simulink subsystem "ACDCConveter"  (R2024a)
settings: Solver=VariableStepAuto  StartTime=0.0  StopTime=1.5  RelTol=1e-3
undefined symbols (not defined in the file): D1, Delta, DiscIntNeverNeededParam, Ts_Control, Ts_Power
libraries: spsSeriesRLCBranchLib x5, spsSecondOrderFilterLib x3, spsThreePhaseSeriesRLCLoadLib x2, spsMeanLib x2, spsabctodq0Lib x2, spsVoltageMeasurementLib x2, spsStairGeneratorLib x1, spsThreePhaseVIMeasurementLib x1, spsPLL3phLib x1, simulink_extras x1, spsPWMGenerator3LevelLib x1, spsGroundLib x1
settings Model: DefaultTestHarness=ACDCConveter_Harness1  Creator=nakamura  LastModifiedBy=nakamura

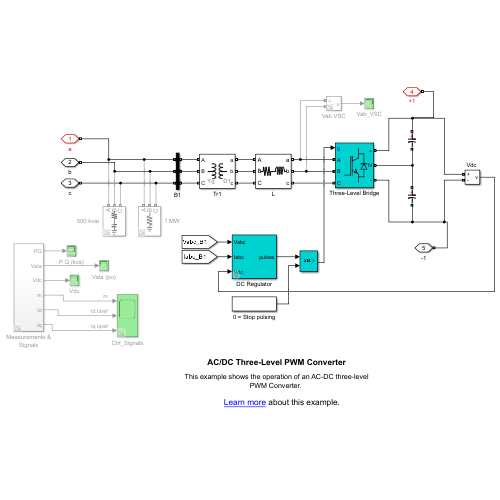
[thumbnail: Simulink's stored preview of the top-level diagram]
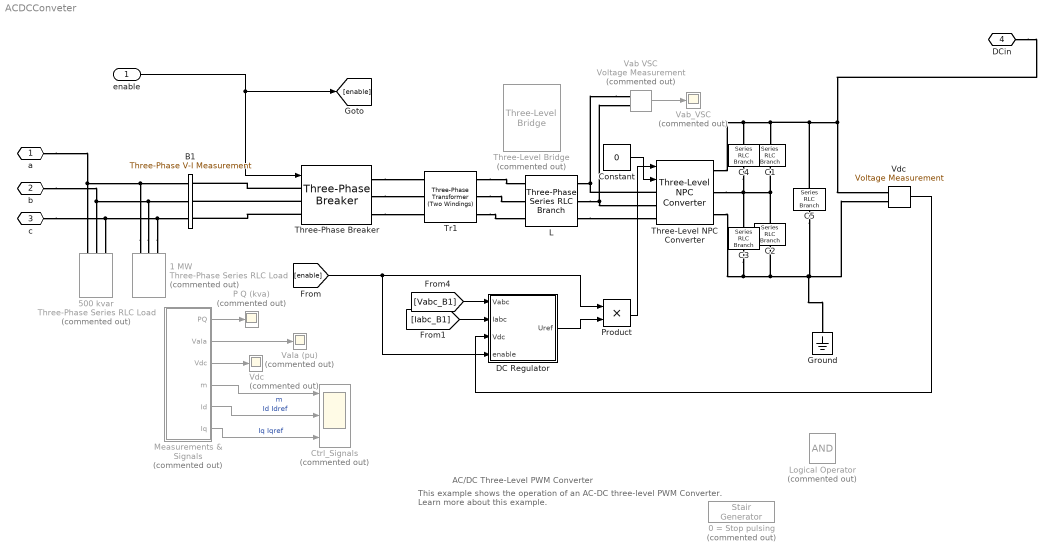
== system ACDCConveter ==
  note: AC/DC Three-Level PWM Converter
  note: This example shows the operation of an AC-DC three-level PWM Converter.
      |
      | Learn more about this example.
  enable : Inport
  0 = Stop pulsing : spsStairGeneratorLib/Stair Generator  Commented=on  t=[0 0.1]*10000000  e=[1 0]  Ts=Ts_Power
  1 MW : spsThreePhaseSeriesRLCLoadLib/Three-Phase Series RLC Load  Commented=on  LConnTagsString=A|B|C  Configuration=Y (grounded)  NominalVoltage=600  Vabc=[1e3 1e3 1e3]  Vabcp=[1e3 1e3 1e3]  NominalFrequency=60  UnbalancedPower=off  ActivePower=1e6  InductivePower=0  CapacitivePower=0  Pabc=[10e3 9e3 11e3]  QLabc=[100 90 110]  QCabc=[100 90 110]  Pabcp=[10e3 9e3 11e3]  QLabcp=[100 90 110]  QCabcp=[100 90 110]  Measurements=None  LoadType=constant Z
  500 kvar : spsThreePhaseSeriesRLCLoadLib/Three-Phase Series RLC Load  Commented=on  LConnTagsString=A|B|C  Configuration=Y (grounded)  NominalVoltage=600  Vabc=[1e3 1e3 1e3]  Vabcp=[1e3 1e3 1e3]  NominalFrequency=60  UnbalancedPower=off  ActivePower=0.5e6/100  InductivePower=0  CapacitivePower=0.5e6  Pabc=[10e3 9e3 11e3]  QLabc=[100 90 110]  QCabc=[100 90 110]  Pabcp=[10e3 9e3 11e3]  QLabcp=[100 90 110]  QCabcp=[100 90 110]  Measurements=None  LoadType=constant Z
  B1 : spsThreePhaseVIMeasurementLib/Three-Phase V-I Measurement  VoltageMeasurement=phase-to-ground  SetLabelV=on  LabelV=Vabc_B1  Vpu=off  VpuLL=off  CurrentMeasurement=yes  SetLabelI=on  LabelI=Iabc_B1  Ipu=off  Pbase=100e6  Vbase=500e3  OutputType=Magnitude  PhasorSimulation=off  PSBequivalent=0
  C1 : spsSeriesRLCBranchLib/Series RLC Branch  LConnTagsString=__new0  RConnTagsString=__new0  BranchType=C  Resistance=1.0  Inductance=1.0  SetiL0=off  InitialCurrent=0  Capacitance=75000e-06  Setx0=off  InitialVoltage=0  Measurements=None
  C2 : spsSeriesRLCBranchLib/Series RLC Branch  LConnTagsString=__new0  RConnTagsString=__new0  BranchType=C  Resistance=1.0  Inductance=1.0  SetiL0=off  InitialCurrent=0  Capacitance=75000e-06  Setx0=off  InitialVoltage=0  Measurements=None
  C3 : spsSeriesRLCBranchLib/Series RLC Branch  LConnTagsString=__new0  RConnTagsString=__new0  BranchType=R  Resistance=1e8  Inductance=1.0  SetiL0=off  InitialCurrent=0  Capacitance=75000e-06  Setx0=off  InitialVoltage=0  Measurements=None
  C4 : spsSeriesRLCBranchLib/Series RLC Branch  LConnTagsString=__new0  RConnTagsString=__new0  BranchType=R  Resistance=1e8  Inductance=1.0  SetiL0=off  InitialCurrent=0  Capacitance=75000e-06  Setx0=off  InitialVoltage=0  Measurements=None
  C5 : spsSeriesRLCBranchLib/Series RLC Branch  LConnTagsString=__new0  RConnTagsString=__new0  BranchType=C  Resistance=1.0  Inductance=1.0  SetiL0=off  InitialCurrent=0  Capacitance=1e-03  Setx0=off  InitialVoltage=0  Measurements=None
  Constant : Constant  Value=0
  Ctrl_Signals : Scope  Commented=on  NumInputPorts=3
  DC Regulator : Subsystem  mask(DC Voltage Regulator){Vdc_Ref=450}
      mask prompts: Vdc_Ref "DC voltage setpoint (V):"
  Ground : spsGroundLib/Ground  LConnTagsString=a
  L : spsThreePhaseSeriesRLCBranchLib/Three-Phase Series RLC Branch  LConnTagsString=A|B|C  RConnTagsString=A|B|C  BranchType=RL  Resistance=0.1e-3  Inductance=20e-6  Capacitance=inf  Measurements=None
  Logical Operator : Logic  Commented=on  AllPortsSameDT=off  OutDataTypeStr=float('double')
  Measurements & Signals : Subsystem  Commented=on
  P Q (kva) : Scope  Commented=on
  Product : Product
  Three-Level NPC Converter : spsThreeLevelNPCConverterLib/Three-Level NPC Converter  ModelType=Average model (Uref-controlled)  Ron=1e-7  Rs=1e6  Cs=inf  Vforward=[0,0]  Ron_Diode=1e-6  Rs_Diode=1e6  Cs_Diode=inf  Vf_Diode=0  Rs_CurrentSource=inf  Ron_ACsource=1e-10
  Three-Level Bridge : spsThreeLevelBridgeLib/Three-Level Bridge  Commented=on  Arms=3  SnubberResistance=50  SbubberCapacitance=1e-6  Device=IGBT / Diodes  Ron=0.2e-3  ForwardVoltages="[  2 1 ]"  Measurements=All voltages and currents
      settings: AttributesFormatString=\n
  Three-Phase Breaker : spsThreePhaseBreakerLib/Three-Phase Breaker  InitialState=open  SwitchA=on  SwitchB=on  SwitchC=on  SwitchTimes="[1/60  5/60]"  External=on  BreakerResistance=1e-6  SnubberResistance=1e7  SnubberCapacitance=inf  Measurements=None
  Tr1 : spsThreePhaseTransformerTwoWindingsLib/Three-Phase Transformer (Two Windings)  Winding1Connection=Yg  Winding2Connection=Delta (D1)  CoreType=Three single-phase transformers  SetSaturation=off  Hysteresis=off  DataFile='hysteresis'  SetInitialFlux=off  Measurements=None  UNITS=pu  NominalPower=[ 500e3 , 60 ]  Winding1=[ 6.6e3 , 0.04/30/2 , 0.04 ]  Winding2=[ 210 , 0.04/30/2 , 0.0 ]  Rm=500  Lm=500  L0=0.5  Saturation=[ 0,0 ; 0.0024,1.2 ; 1.0,1.52 ]  InitialFluxes=[ 0.8 , -0.8 , 0.7 ]  BreakLoop=off  DiscreteSolver=Trapezoidal iterative  DataType=off  TransfoNumber=0
  VaIa (pu) : Scope  Commented=on
  Vab VSC : spsVoltageMeasurementLib/Voltage Measurement  Tag=PoWeRsYsTeMmEaSuReMeNt  Commented=on  PhasorSimulation=off  OutputType=Magnitude  PSBequivalent=0
  Vab_VSC : Scope  Commented=on
  Vdc : Scope  Commented=on
  "Vdc " : spsVoltageMeasurementLib/Voltage Measurement  Tag=PoWeRsYsTeMmEaSuReMeNt  PhasorSimulation=off  OutputType=Magnitude  PSBequivalent=0
  a : PMIOPort  Side=Left
  b : PMIOPort  Port=2  Side=Left
  c : PMIOPort  Port=3  Side=Left
  DCin : PMIOPort  Port=4  Side=Right
  wires:
  Measurements & Signals/5(Id) -> Ctrl_Signals/2  "Id Idref"
  Measurements & Signals/6(Iq) -> Ctrl_Signals/3  "Iq Iqref"
  [Iabc_B1] -> DC Regulator/2(Iabc)
  Measurements & Signals/4(m) -> Ctrl_Signals/1  "m"
  Measurements & Signals/1(PQ) -> P Q (kva)/1
  Vab VSC/1 -> Vab_VSC/1
  Measurements & Signals/2(VaIa) -> VaIa (pu)/1
  [Vabc_B1] -> DC Regulator/1(Vabc)
  "Vdc "/1 -> DC Regulator/3(Vdc)
  Measurements & Signals/3(Vdc) -> Vdc/1
  Constant/1 -> Three-Level NPC Converter/2
  Product/1 -> Three-Level NPC Converter/1
  enable/1 -> [enable], Three-Phase Breaker/1
  [enable] -> Product/1, DC Regulator/4(enable)
  DC Regulator/1(Uref) -> Product/2
  connections:
  1 MW/LConn1 -- a/RConn1 -- 500 kvar/LConn1 -- B1/LConn1
  C5/RConn1 -- "Vdc "/LConn2 -- Ground/LConn1 -- Three-Level NPC Converter/RConn3 -- C3/RConn1 -- C2/RConn1
  Three-Level NPC Converter/RConn1 -- C4/LConn1 -- C1/LConn1 -- C5/LConn1 -- "Vdc "/LConn1 -- DCin/RConn1
  C2/LConn1 -- Three-Level NPC Converter/RConn2 -- C4/RConn1 -- C3/LConn1 -- C1/RConn1
  1 MW/LConn3 -- c/RConn1 -- 500 kvar/LConn3 -- B1/LConn3
  1 MW/LConn2 -- b/RConn1 -- 500 kvar/LConn2 -- B1/LConn2
  L/RConn2 -- Vab VSC/LConn2 -- Three-Level NPC Converter/LConn2
  Vab VSC/LConn1 -- Three-Level NPC Converter/LConn1 -- L/RConn1
  Three-Phase Breaker/LConn2 -- B1/RConn2
  Three-Phase Breaker/LConn3 -- B1/RConn3
  Tr1/RConn1 -- L/LConn1
  Three-Phase Breaker/LConn1 -- B1/RConn1
  Tr1/RConn3 -- L/LConn3
  L/RConn3 -- Three-Level NPC Converter/LConn3
  Tr1/RConn2 -- L/LConn2
  Three-Phase Breaker/RConn1 -- Tr1/LConn1
  Three-Phase Breaker/RConn2 -- Tr1/LConn2
  Three-Phase Breaker/RConn3 -- Tr1/LConn3

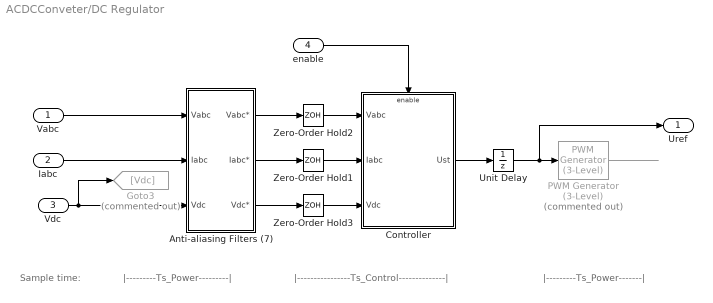
== system ACDCConveter/DC Regulator ==
  note: |----------------Ts_Control--------------|
  note: |---------Ts_Power---------|
  note: Sample time:
  note: |---------Ts_Power-------|
  Vabc : Inport  PortDimensions=3
  Iabc : Inport  Port=2  PortDimensions=3
  Vdc : Inport  Port=3  PortDimensions=1
  enable : Inport  Port=4  PortDimensions=1
  Anti-aliasing Filters (7) : Subsystem  mask(Anti-aliasing (2nd order lowpass)){Fc=750, Ts=Ts_Power}
      mask prompts: Fc "Cut-off frequency (Hz):"; Ts "Sample time:"
  Controller : Subsystem  mask(DC Regulator){Vdc_Ref=Vdc_Ref, Par_VdcReg=[0.015 1.6], Par_IReg=[0.3 20], Par_Nom=[6.6e3 500e3], Ts=Ts_Control}
      mask prompts: Vdc_Ref "DC Voltage setpoint (Volts)"; Par_VdcReg "Vdc Regulator Gains: [ Kp  Ki ]"; Par_IReg "Current Regulators Gain: [ Kp Ki Kd ]"; Par_Nom "Nominal Voltage and power: [ Vnom (volts rms L-L)  Pnom (VA) ]"; Ts "Time Step (s)"
      mask init:
      | Vnom=Par_Nom(1);
      | Pnom=Par_Nom(2);
      | Kp_I=Par_IReg(1);
      | Ki_I=Par_IReg(2);
      | Kp_Vdc=Par_VdcReg(1);
      | Ki_Vdc=Par_VdcReg(2);
  Goto3 : Goto  Commented=on  GotoTag=Vdc
  PWM Generator (3-Level) : spsPWMGenerator3LevelLib/PWM Generator (3-Level)  Commented=on  ModulatorType=Three-phase bridge (12 pulses)  ModulatorMode=Unsynchronized  nF=27  Fc=27*60  ModulatingSignals=off  m=0.8  Freq=60  Phase=0  Ts=Ts_Power
  Unit Delay : UnitDelay  SampleTime=Ts_Control  HasFrameUpgradeWarning=on
  Zero-Order Hold1 : ZeroOrderHold  SampleTime=Ts_Control
  Zero-Order Hold2 : ZeroOrderHold  SampleTime=Ts_Control
  Zero-Order Hold3 : ZeroOrderHold  SampleTime=Ts_Control
  Uref : Outport  VectorParamsAs1DForOutWhenUnconnected=off
  wires:
  enable/1 -> Controller/Enable
  PWM Generator (3-Level)/1 -> ?
  Unit Delay/1 -> PWM Generator (3-Level)/1, Uref/1
  Controller/1(Ust) -> Unit Delay/1
  Anti-aliasing Filters (7)/1(" Vabc*") -> Zero-Order Hold2/1
  Anti-aliasing Filters (7)/2(Iabc*) -> Zero-Order Hold1/1
  Anti-aliasing Filters (7)/3(" Vdc*") -> Zero-Order Hold3/1
  Zero-Order Hold3/1 -> Controller/3(Vdc)
  Zero-Order Hold1/1 -> Controller/2(Iabc)
  Zero-Order Hold2/1 -> Controller/1(Vabc)
  Vdc/1 -> Goto3/1, Anti-aliasing Filters (7)/3("Vdc ")
  Iabc/1 -> Anti-aliasing Filters (7)/2("Iabc ")
  Vabc/1 -> Anti-aliasing Filters (7)/1(Vabc)

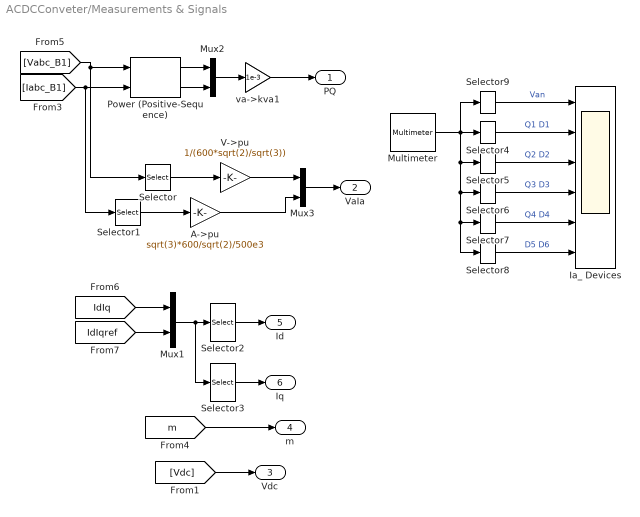
== system ACDCConveter/Measurements & Signals ==
  A->pu : Gain  Gain=sqrt(3)*600/sqrt(2)/500e3  SaturateOnIntegerOverflow=on  OutDataTypeStr=Inherit: Same as input  ParamDataTypeStr=Inherit: Same as input
  Ia_ Devices : Scope  NumInputPorts=6
  Multimeter : spsMultimeterLib/Multimeter  Tag=PoWeRsYsTeMmEaSuReMeNt  L=35  sel=[1 6 7 8 9 10 11 12 13 14 15]  yselected={}  Gain=[1 1 1 1 1 1 1 1 1 1 1]  OutputType=Magnitude  PlotAtSimulationStop=off  PhasorSimulation=off
      settings: AttributesFormatString=\n
  Mux1 : Mux  Inputs=2
  Mux2 : Mux  Inputs=2
  Mux3 : Mux  Inputs=2
  Power (Positive-Sequence) : spsPowerPositiveSequenceLib/Power (Positive-Sequence)  Freq=60  Vinit=[370 0]  Iinit=[5 0]  Ts=Ts_Power
  Selector : Selector  InputPortWidth=3  IndexOptions=Index vector (dialog)  Indices=1  OutputSizes=1
  Selector1 : Selector  InputPortWidth=3  IndexOptions=Index vector (dialog)  Indices=1  OutputSizes=1
  Selector2 : Selector  InputPortWidth=4  IndexOptions=Index vector (dialog)  Indices=[1 3]  OutputSizes=1
  Selector3 : Selector  InputPortWidth=4  IndexOptions=Index vector (dialog)  Indices=[1 3]+1  OutputSizes=1
  Selector4 : Selector  InputPortWidth=11  IndexOptions=Index vector (dialog)  Indices=[1 5]+1  OutputSizes=1
  Selector5 : Selector  InputPortWidth=11  IndexOptions=Index vector (dialog)  Indices=[1 5]+2  OutputSizes=1
  Selector6 : Selector  InputPortWidth=11  IndexOptions=Index vector (dialog)  Indices=[1 5]+3  OutputSizes=1
  Selector7 : Selector  InputPortWidth=11  IndexOptions=Index vector (dialog)  Indices=[1 5]+4  OutputSizes=1
  Selector8 : Selector  InputPortWidth=11  IndexOptions=Index vector (dialog)  Indices=[10 11]  OutputSizes=1
  Selector9 : Selector  InputPortWidth=11  IndexOptions=Index vector (dialog)  Indices=1  OutputSizes=1
  V->pu : Gain  Gain=1/(600*sqrt(2)/sqrt(3))  SaturateOnIntegerOverflow=on  OutDataTypeStr=Inherit: Same as input  ParamDataTypeStr=Inherit: Same as input
  va->kva1 : Gain  Gain=1e-3  SaturateOnIntegerOverflow=on  OutDataTypeStr=Inherit: Same as input  ParamDataTypeStr=Inherit: Same as input
  PQ : Outport  VectorParamsAs1DForOutWhenUnconnected=off
  VaIa : Outport  Port=2  VectorParamsAs1DForOutWhenUnconnected=off
  Vdc : Outport  Port=3  VectorParamsAs1DForOutWhenUnconnected=off
  m : Outport  Port=4  VectorParamsAs1DForOutWhenUnconnected=off
  Id : Outport  Port=5  VectorParamsAs1DForOutWhenUnconnected=off
  Iq : Outport  Port=6  VectorParamsAs1DForOutWhenUnconnected=off
  wires:
  Selector8/1 -> Ia_ Devices/6  "D5 D6"
  Selector7/1 -> Ia_ Devices/5  "Q4 D4"
  Selector6/1 -> Ia_ Devices/4  "Q3 D3"
  Selector5/1 -> Ia_ Devices/3  "Q2 D2"
  Selector4/1 -> Ia_ Devices/2  "Q1 D1"
  Selector9/1 -> Ia_ Devices/1  "Van"
  A->pu/1 -> Mux3/2
  V->pu/1 -> Mux3/1
  Selector3/1 -> Iq/1
  Selector2/1 -> Id/1
  [m] -> m/1
  Mux1/1 -> Selector3/1, Selector2/1
  [Vdc] -> Vdc/1
  Mux3/1 -> VaIa/1
  [Iabc_B1] -> Power (Positive-Sequence)/2, Selector1/1
  [Vabc_B1] -> Power (Positive-Sequence)/1, Selector/1
  Selector1/1 -> A->pu/1
  Selector/1 -> V->pu/1
  [IdIqref] -> Mux1/2
  [IdIq] -> Mux1/1
  Multimeter/1 -> Selector9/1, Selector8/1, Selector7/1, Selector6/1, Selector5/1, Selector4/1
  Power (Positive-Sequence)/1 -> Mux2/1
  Power (Positive-Sequence)/2 -> Mux2/2
  Mux2/1 -> va->kva1/1
  va->kva1/1 -> PQ/1

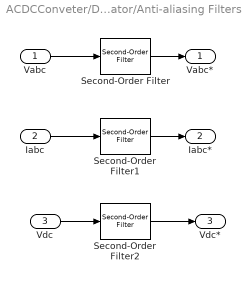
== system ACDCConveter/DC Regulator/Anti-aliasing Filters (7) ==
  Vabc : Inport  PortDimensions=3
  "Iabc " : Inport  Port=2  PortDimensions=3
  "Vdc " : Inport  Port=3  PortDimensions=1
  Second-Order Filter : spsSecondOrderFilterLib/Second-Order Filter  FilterType=Lowpass  Fo=Fc  Zeta=0.707  Ts=Ts  Initialize=off  Vac_Init="[0,  0,  60]"  Vdc_Init=0  PlotResponse=off  FreqRange=[0, 500, 1]
  Second-Order Filter1 : spsSecondOrderFilterLib/Second-Order Filter  FilterType=Lowpass  Fo=Fc  Zeta=0.707  Ts=Ts  Initialize=off  Vac_Init="[0,  0,  60]"  Vdc_Init=0  PlotResponse=off  FreqRange=[0, 500, 1]
  Second-Order Filter2 : spsSecondOrderFilterLib/Second-Order Filter  FilterType=Lowpass  Fo=Fc  Zeta=0.707  Ts=Ts  Initialize=off  Vac_Init="[0,  0,  60]"  Vdc_Init=0  PlotResponse=off  FreqRange=[0, 500, 1]
  " Vabc*" : Outport  VectorParamsAs1DForOutWhenUnconnected=off
  Iabc* : Outport  Port=2  VectorParamsAs1DForOutWhenUnconnected=off
  " Vdc*" : Outport  Port=3  VectorParamsAs1DForOutWhenUnconnected=off
  wires:
  Second-Order Filter2/1 -> " Vdc*"/1
  "Vdc "/1 -> Second-Order Filter2/1
  Vabc/1 -> Second-Order Filter/1
  Second-Order Filter/1 -> " Vabc*"/1
  "Iabc "/1 -> Second-Order Filter1/1
  Second-Order Filter1/1 -> Iabc*/1

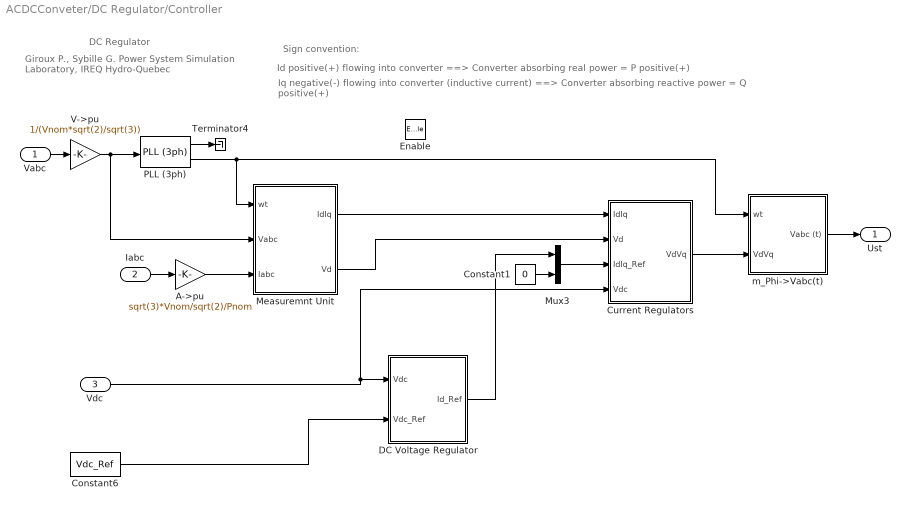
== system ACDCConveter/DC Regulator/Controller ==
  note: DC Regulator
  note: Giroux P., Sybille G.
      | Power System Simulation Laboratory, IREQ
      | Hydro-Quebec
  note: Iq negative(-) flowing into converter (inductive current) ==> Converter absorbing reactive power = Q positive(+)
  note: Sign convention:
  note: Id positive(+) flowing into converter ==> Converter absorbing real power = P positive(+)
  Vabc : Inport  PortDimensions=3
  Iabc : Inport  Port=2  PortDimensions=3
  Vdc : Inport  Port=3  PortDimensions=1
  Enable : EnablePort  StatesWhenEnabling=reset
  A->pu : Gain  Gain=sqrt(3)*Vnom/sqrt(2)/Pnom  SaturateOnIntegerOverflow=on  OutDataTypeStr=Inherit: Same as input  ParamDataTypeStr=Inherit: Same as input
  Constant1 : Constant  Value=0
  Constant6 : Constant  Value=Vdc_Ref
  Current Regulators : Subsystem  mask(Current Regulators){Kp=Kp_I, Ki=Ki_I, Kd=0, TcD=0.2e-3, Par_Limits=[12 -12], Init=0, Ts=Ts}
      mask prompts: Kp "Proportional gain (Kp):"; Ki "Integral gain (Ki):"; Kd "Derivative gain (Kd):"; TcD "Time constant for derivative (s):"; Par_Limits "Output limits: [ Upper   Lower ]"; Init "Output initial value:"; Ts "Sample time:"
      mask help:
      | Sign convention:
      | Id positive(+) flowing into converter ==> Converter absorbing real power = P positive(+)
      | Iq negative(-) flowing into converter (inductive current) ==> Converter absorbing reactive power = Q positive(+)
  DC Voltage Regulator : Subsystem  mask(DC Voltage regulator){Kp=Kp_Vdc, Ki=Ki_Vdc, Ts=Ts}
      mask prompts: Kp "Proportional gain (Kp):"; Ki "Integral gain(Ki)"; Ts "Sample time:"
  Measuremnt Unit : Subsystem
  Mux3 : Mux  Inputs=2
  PLL (3ph) : spsPLL3phLib/PLL (3ph)  Fmin=45  Par_Init=[-45 60]  ParK=[60 1400]  TcD=1e-4  MaxRateChangeFreq=12  FilterCutOffFreq=25  Ts=1e-5  AGC=off
  Terminator4 : Terminator
  V->pu : Gain  Gain=1/(Vnom*sqrt(2)/sqrt(3))  SaturateOnIntegerOverflow=on  OutDataTypeStr=Inherit: Same as input  ParamDataTypeStr=Inherit: Same as input
  m_Phi->Vabc(t) : Subsystem
  Ust : Outport  VectorParamsAs1DForOutWhenUnconnected=off
  wires:
  Constant6/1 -> DC Voltage Regulator/2(Vdc_Ref)
  m_Phi->Vabc(t)/1(Vabc (t)) -> Ust/1
  PLL (3ph)/2 -> m_Phi->Vabc(t)/1(wt), Measuremnt Unit/1(wt)
  Current Regulators/1(VdVq) -> m_Phi->Vabc(t)/2(VdVq)
  DC Voltage Regulator/1(Id_Ref) -> Mux3/1
  Constant1/1 -> Mux3/2
  Mux3/1 -> Current Regulators/3(IdIq_Ref)
  Measuremnt Unit/2(Vd) -> Current Regulators/2(Vd)
  Measuremnt Unit/1(IdIq) -> Current Regulators/1(IdIq)
  Iabc/1 -> A->pu/1
  PLL (3ph)/1 -> Terminator4/1
  Vdc/1 -> Current Regulators/4(Vdc), DC Voltage Regulator/1(Vdc)
  Vabc/1 -> V->pu/1
  V->pu/1 -> PLL (3ph)/1, Measuremnt Unit/2(Vabc)
  A->pu/1 -> Measuremnt Unit/3(Iabc)

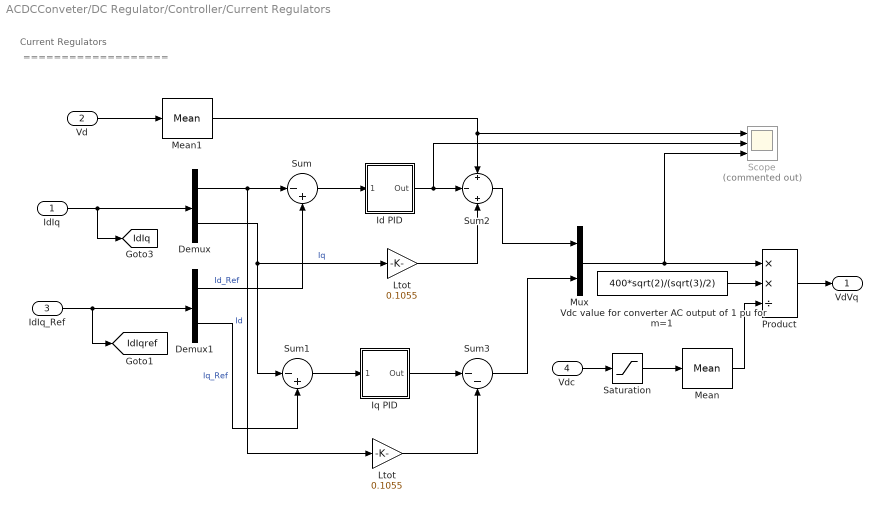
== system ACDCConveter/DC Regulator/Controller/Current Regulators ==
  note: ===================
  note: Current Regulators
  IdIq : Inport  PortDimensions=2
  Vd : Inport  Port=2
  IdIq_Ref : Inport  Port=3  PortDimensions=2
  Vdc : Inport  Port=4
  " Ltot" : Gain  Gain=0.1055  SaturateOnIntegerOverflow=on  OutDataTypeStr=Inherit: Same as input  ParamDataTypeStr=Inherit: Same as input
  Demux : Demux  Outputs=2
      settings: DisplayOption=none
  Demux1 : Demux  Outputs=2
      settings: DisplayOption=none
  Id PID : Subsystem  DialogController=POWERSYS.PowerSysDialog  mask(Discrete PID Controller){Kp=Kp, Ki=Ki, Kd=Kd, TcD=TcD, Par_Limits=Par_Limits, Init=Init, Ts=Ts}
      mask prompts: Kp "Proportional gain (Kp):"; Ki "Integral gain (Ki):"; Kd "Derivative gain (Kd):"; TcD "Time constant for derivative (s):"; Par_Limits "Output limits: [ Upper   Lower ]"; Init "Output initial value:"; Ts "Sample time:"
      mask help: This block implements a discrete PID controller.
      mask init:
      | UpperLimit=Par_Limits(1);
      | LowerLimit=Par_Limits(2);
      | power_initmask();
      mask Display: disp('PID');
  Iq PID : Subsystem  DialogController=POWERSYS.PowerSysDialog  mask(Discrete PID Controller){Kp=Kp, Ki=Ki, Kd=Kd, TcD=TcD, Par_Limits=Par_Limits, Init=Init, Ts=Ts}
      mask prompts: Kp "Proportional gain (Kp):"; Ki "Integral gain (Ki):"; Kd "Derivative gain (Kd):"; TcD "Time constant for derivative (s):"; Par_Limits "Output limits: [ Upper   Lower ]"; Init "Output initial value:"; Ts "Sample time:"
      mask help: This block implements a discrete PID controller.
      mask init:
      | UpperLimit=Par_Limits(1);
      | LowerLimit=Par_Limits(2);
      | power_initmask();
      mask Display: disp('PID');
  "Ltot " : Gain  Gain=0.1055  SaturateOnIntegerOverflow=on  OutDataTypeStr=Inherit: Same as input  ParamDataTypeStr=Inherit: Same as input
  Mean : spsMeanLib/Mean  Freq=60  Vinit=500  Ts=Ts
  Mean1 : spsMeanLib/Mean  Freq=60  Vinit=1.007  Ts=Ts
  Mux : Mux  Inputs=2
  Product : Product  Inputs=**/  InputSameDT=on  SaturateOnIntegerOverflow=on  OutDataTypeStr=Inherit: Same as first input
  Saturation : Saturate  UpperLimit=10000  LowerLimit=10
  Scope : Scope  Commented=on  NumInputPorts=3
  Sum : Sum  Inputs=|-+  InputSameDT=on  SaturateOnIntegerOverflow=on  OutDataTypeStr=Inherit: Same as first input
  Sum1 : Sum  Inputs=|-+  InputSameDT=on  SaturateOnIntegerOverflow=on  OutDataTypeStr=Inherit: Same as first input
  Sum2 : Sum  Inputs=+|-|+  InputSameDT=on  SaturateOnIntegerOverflow=on  OutDataTypeStr=Inherit: Same as first input
  Sum3 : Sum  Inputs=|--  InputSameDT=on  SaturateOnIntegerOverflow=on  OutDataTypeStr=Inherit: Same as first input
  Vdc value for converter AC output of 1 pu for m=1 : Constant  Value=400*sqrt(2)/(sqrt(3)/2)
  VdVq : Outport  VectorParamsAs1DForOutWhenUnconnected=off
  tag scope: IdIq=global, IdIqref=global
  wires:
  Sum3/1 -> Mux/2
  Vdc/1 -> Saturation/1
  Mean/1 -> Product/3
  Vdc value for converter AC output of 1 pu for m=1/1 -> Product/2
  Saturation/1 -> Mean/1
  Mean1/1 -> Scope/1, Sum2/1
  Product/1 -> VdVq/1
  IdIq_Ref/1 -> [IdIqref], Demux1/1
  Mux/1 -> Scope/3, Product/1
  Sum/1 -> Id PID/1(Error)
  Demux1/2 -> Sum1/2  "Iq_Ref"
  Sum1/1 -> Iq PID/1(Error)
  Demux/2 -> Sum1/1, "Ltot "/1  "Iq"
  Demux1/1 -> Sum/2  "Id_Ref"
  Demux/1 -> " Ltot"/1, Sum/1  "Id"
  IdIq/1 -> [IdIq], Demux/1
  Id PID/1(Out) -> Scope/2, Sum2/2
  Sum2/1 -> Mux/1
  Iq PID/1(Out) -> Sum3/1
  "Ltot "/1 -> Sum2/3
  " Ltot"/1 -> Sum3/2
  Vd/1 -> Mean1/1

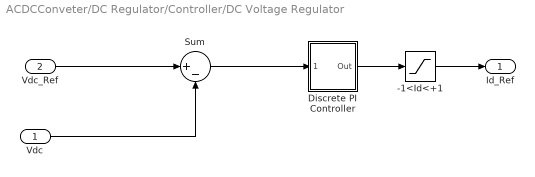
== system ACDCConveter/DC Regulator/Controller/DC Voltage Regulator ==
  Vdc : Inport
  Vdc_Ref : Inport  Port=2
  -1<Id<+1 : Saturate  UpperLimit=1.2  LowerLimit=-1.2
  Discrete PI Controller : Subsystem  DialogController=POWERSYS.PowerSysDialog  mask(Discrete PI Controller){Kp=Kp, Ki=Ki, Par_Limits=[1.2 -1.2]*10, Init=0, Ts=Ts}
      mask prompts: Kp "Proportional gain (Kp):"; Ki "Integral gain (Ki):"; Par_Limits "Output limits: [ Upper   Lower ]"; Init "Output initial value:"; Ts "Sample time:"
      mask help: This block implements a discrete PI controller.
      mask init:
      | UpperLimit=Par_Limits(1);
      | LowerLimit=Par_Limits(2);
      | power_initmask();
      mask Display: disp('PI');
  Sum : Sum  Inputs=|+-  InputSameDT=on  SaturateOnIntegerOverflow=on  OutDataTypeStr=Inherit: Same as first input
  Id_Ref : Outport  InitialOutput=0  VectorParamsAs1DForOutWhenUnconnected=off
  wires:
  Sum/1 -> Discrete PI Controller/1(Error)
  Vdc/1 -> Sum/2
  Discrete PI Controller/1(Out) -> -1<Id<+1/1
  -1<Id<+1/1 -> Id_Ref/1
  Vdc_Ref/1 -> Sum/1

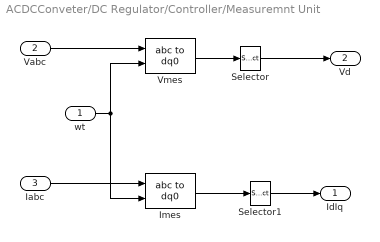
== system ACDCConveter/DC Regulator/Controller/Measuremnt Unit ==
  wt : Inport
  Vabc : Inport  Port=2
  Iabc : Inport  Port=3
  Imes : spsabctodq0Lib/abc to dq0  Alignment=90 degrees behind phase A axis
  Selector : Selector  InputPortWidth=3  IndexOptions=Index vector (dialog)  Indices=1  OutputSizes=1
  Selector1 : Selector  InputPortWidth=3  IndexOptions=Index vector (dialog)  Indices=[1 2]  OutputSizes=1
  Vmes : spsabctodq0Lib/abc to dq0  Alignment=90 degrees behind phase A axis
  IdIq : Outport  VectorParamsAs1DForOutWhenUnconnected=off
  Vd : Outport  Port=2  VectorParamsAs1DForOutWhenUnconnected=off
  wires:
  Selector/1 -> Vd/1
  Imes/1 -> Selector1/1
  Iabc/1 -> Imes/1
  wt/1 -> Imes/2, Vmes/2
  Vmes/1 -> Selector/1
  Vabc/1 -> Vmes/1
  Selector1/1 -> IdIq/1

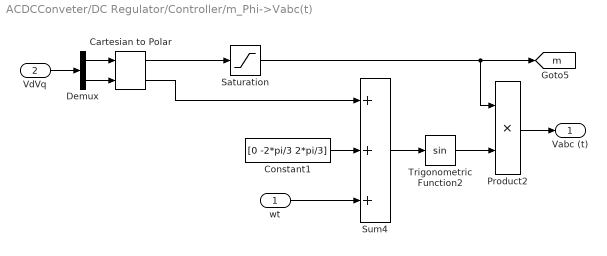
== system ACDCConveter/DC Regulator/Controller/m_Phi->Vabc(t) ==
  wt : Inport
  VdVq : Inport  Port=2
  Cartesian to Polar : simulink_extras/Transformations/Cartesian to Polar
  Constant1 : Constant  Value=[0 -2*pi/3 2*pi/3]
  Demux : Demux  Outputs=2
      settings: DisplayOption=none
  Product2 : Product  InputSameDT=on  SaturateOnIntegerOverflow=on  OutDataTypeStr=Inherit: Same as first input
  Saturation : Saturate  UpperLimit=1  LowerLimit=0
  Sum4 : Sum  Inputs=+++  InputSameDT=on  SaturateOnIntegerOverflow=on  OutDataTypeStr=Inherit: Same as first input
  Trigonometric Function2 : Trigonometry
  Vabc (t) : Outport  VectorParamsAs1DForOutWhenUnconnected=off
  tag scope: m=global
  wires:
  Saturation/1 -> [m], Product2/1
  Cartesian to Polar/1 -> Saturation/1
  Trigonometric Function2/1 -> Product2/2
  Sum4/1 -> Trigonometric Function2/1
  Cartesian to Polar/2 -> Sum4/1
  Demux/2 -> Cartesian to Polar/2
  Demux/1 -> Cartesian to Polar/1
  VdVq/1 -> Demux/1
  wt/1 -> Sum4/3
  Product2/1 -> Vabc (t)/1
  Constant1/1 -> Sum4/2

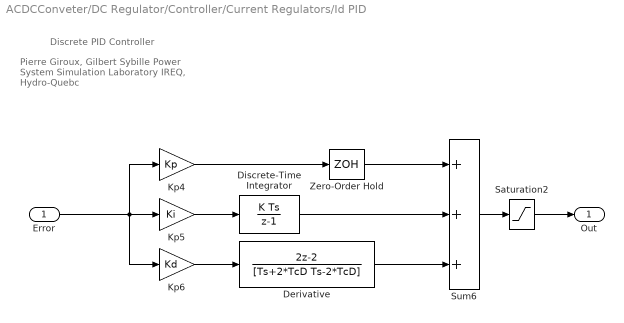
== system ACDCConveter/DC Regulator/Controller/Current Regulators/Id PID ==
  note: Pierre Giroux, Gilbert Sybille
      | Power System Simulation Laboratory
      | IREQ, Hydro-Quebc
  note: Discrete PID Controller
  Error : Inport  SampleTime=Ts
  "Derivative " : DiscreteTransferFcn  Numerator=[2 -2]  Denominator=[Ts+2*TcD Ts-2*TcD]  SampleTime=Ts
  Discrete-Time Integrator : DiscreteIntegrator  InitialCondition=Init  SampleTime=Ts  LimitOutput=on  UpperSaturationLimit=UpperLimit  LowerSaturationLimit=LowerLimit  ICPrevOutput=DiscIntNeverNeededParam  ICPrevScaledInput=DiscIntNeverNeededParam
  Kp4 : Gain  Gain=Kp  SaturateOnIntegerOverflow=on  SampleTime=Ts  OutDataTypeStr=Inherit: Same as input  ParamDataTypeStr=Inherit: Same as input
  Kp5 : Gain  Gain=Ki  SaturateOnIntegerOverflow=on  SampleTime=Ts  OutDataTypeStr=Inherit: Same as input  ParamDataTypeStr=Inherit: Same as input
  Kp6 : Gain  Gain=Kd  SaturateOnIntegerOverflow=on  SampleTime=Ts  OutDataTypeStr=Inherit: Same as input  ParamDataTypeStr=Inherit: Same as input
  Saturation2 : Saturate  UpperLimit=UpperLimit  LowerLimit=LowerLimit  SampleTime=Ts
  Sum6 : Sum  Inputs=+++  InputSameDT=on  SaturateOnIntegerOverflow=on  SampleTime=Ts  OutDataTypeStr=Inherit: Same as first input
  Zero-Order Hold : ZeroOrderHold  SampleTime=Ts
  Out : Outport  SampleTime=Ts  InitialOutput=0  VectorParamsAs1DForOutWhenUnconnected=off
  wires:
  Saturation2/1 -> Out/1
  Error/1 -> Kp4/1, Kp5/1, Kp6/1
  Sum6/1 -> Saturation2/1
  Kp5/1 -> Discrete-Time Integrator/1
  Kp6/1 -> "Derivative "/1
  Kp4/1 -> Zero-Order Hold/1
  Discrete-Time Integrator/1 -> Sum6/2
  "Derivative "/1 -> Sum6/3
  Zero-Order Hold/1 -> Sum6/1

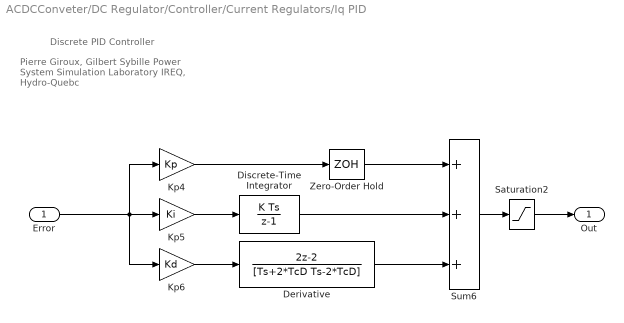
== system ACDCConveter/DC Regulator/Controller/Current Regulators/Iq PID ==
  note: Pierre Giroux, Gilbert Sybille
      | Power System Simulation Laboratory
      | IREQ, Hydro-Quebc
  note: Discrete PID Controller
  Error : Inport  SampleTime=Ts
  "Derivative " : DiscreteTransferFcn  Numerator=[2 -2]  Denominator=[Ts+2*TcD Ts-2*TcD]  SampleTime=Ts
  Discrete-Time Integrator : DiscreteIntegrator  InitialCondition=Init  SampleTime=Ts  LimitOutput=on  UpperSaturationLimit=UpperLimit  LowerSaturationLimit=LowerLimit  ICPrevOutput=DiscIntNeverNeededParam  ICPrevScaledInput=DiscIntNeverNeededParam
  Kp4 : Gain  Gain=Kp  SaturateOnIntegerOverflow=on  SampleTime=Ts  OutDataTypeStr=Inherit: Same as input  ParamDataTypeStr=Inherit: Same as input
  Kp5 : Gain  Gain=Ki  SaturateOnIntegerOverflow=on  SampleTime=Ts  OutDataTypeStr=Inherit: Same as input  ParamDataTypeStr=Inherit: Same as input
  Kp6 : Gain  Gain=Kd  SaturateOnIntegerOverflow=on  SampleTime=Ts  OutDataTypeStr=Inherit: Same as input  ParamDataTypeStr=Inherit: Same as input
  Saturation2 : Saturate  UpperLimit=UpperLimit  LowerLimit=LowerLimit  SampleTime=Ts
  Sum6 : Sum  Inputs=+++  InputSameDT=on  SaturateOnIntegerOverflow=on  SampleTime=Ts  OutDataTypeStr=Inherit: Same as first input
  Zero-Order Hold : ZeroOrderHold  SampleTime=Ts
  Out : Outport  SampleTime=Ts  InitialOutput=0  VectorParamsAs1DForOutWhenUnconnected=off
  wires:
  Saturation2/1 -> Out/1
  Error/1 -> Kp4/1, Kp5/1, Kp6/1
  Sum6/1 -> Saturation2/1
  Kp5/1 -> Discrete-Time Integrator/1
  Kp6/1 -> "Derivative "/1
  Kp4/1 -> Zero-Order Hold/1
  Discrete-Time Integrator/1 -> Sum6/2
  "Derivative "/1 -> Sum6/3
  Zero-Order Hold/1 -> Sum6/1

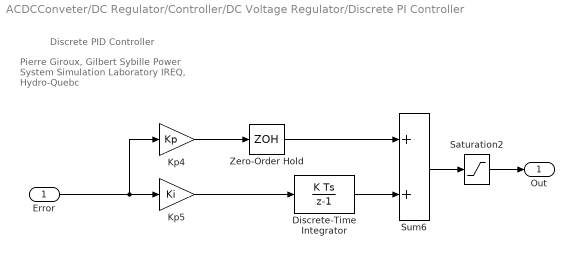
== system ACDCConveter/DC Regulator/Controller/DC Voltage Regulator/Discrete PI Controller ==
  note: Discrete PID Controller
  note: Pierre Giroux, Gilbert Sybille
      | Power System Simulation Laboratory
      | IREQ, Hydro-Quebc
  Error : Inport  SampleTime=Ts
  Discrete-Time Integrator : DiscreteIntegrator  InitialCondition=Init  SampleTime=Ts  LimitOutput=on  UpperSaturationLimit=UpperLimit  LowerSaturationLimit=LowerLimit  ICPrevOutput=DiscIntNeverNeededParam  ICPrevScaledInput=DiscIntNeverNeededParam
  Kp4 : Gain  Gain=Kp  SaturateOnIntegerOverflow=on  SampleTime=Ts  OutDataTypeStr=Inherit: Same as input  ParamDataTypeStr=Inherit: Same as input
  Kp5 : Gain  Gain=Ki  SaturateOnIntegerOverflow=on  SampleTime=Ts  OutDataTypeStr=Inherit: Same as input  ParamDataTypeStr=Inherit: Same as input
  Saturation2 : Saturate  UpperLimit=UpperLimit  LowerLimit=LowerLimit  SampleTime=Ts
  Sum6 : Sum  InputSameDT=on  SaturateOnIntegerOverflow=on  SampleTime=Ts  OutDataTypeStr=Inherit: Same as first input
  Zero-Order Hold : ZeroOrderHold  SampleTime=Ts
  Out : Outport  SampleTime=Ts  InitialOutput=0  VectorParamsAs1DForOutWhenUnconnected=off
  wires:
  Zero-Order Hold/1 -> Sum6/1
  Saturation2/1 -> Out/1
  Discrete-Time Integrator/1 -> Sum6/2
  Kp4/1 -> Zero-Order Hold/1
  Kp5/1 -> Discrete-Time Integrator/1
  Sum6/1 -> Saturation2/1
  Error/1 -> Kp5/1, Kp4/1
